simulink model "drone"  (Simulink 8.5)
settings: Solver=ode45  StartTime=0.0  StopTime=tsim  RelTol=1e-8  AbsTol=1e-12
undefined symbols (not defined in the file or in its folder): A, a_noise_seed, a_noise_var, a_scale, Cd, dx_init, enu2ecef, g, GPS_DT, GuideDt, h_noise_seed, h_noise_var, I, I_motor, IMU_DT, KaQ, KaR, KDhover, KIhover, Kir, KPhover, Kpr, Kpv, KQ, KR, KthQ, KthR, m, mag_bias, MAG_DT, mag_noise_seed, mag_noise_var, MaxPropRate, MaxPwmWidth, mean_a_bias, mean_w_bias, MinPwmWidth, mtow, P_init, Q, q0, qInit, R, r0, r1, r2, r3, r4, r_gps, RateToForce, Re, rho, Rmag, RunUpLimit, RunUpStartThrottle, tc, v0, v_noise_seed, v_noise_var, vc ... (+7)
libraries: simulink x13, SimLib x3
(part 1 of 2)
settings Model: Creator=Mike  LastModifiedBy=Walker  CovSFcnEnable=off
settings SolverCC: ZeroCrossControl=DisableAll
settings DebuggingCC: SolverPrmCheckMsg=warning  FcnCallInpInsideContextMsg=UseLocalSettings

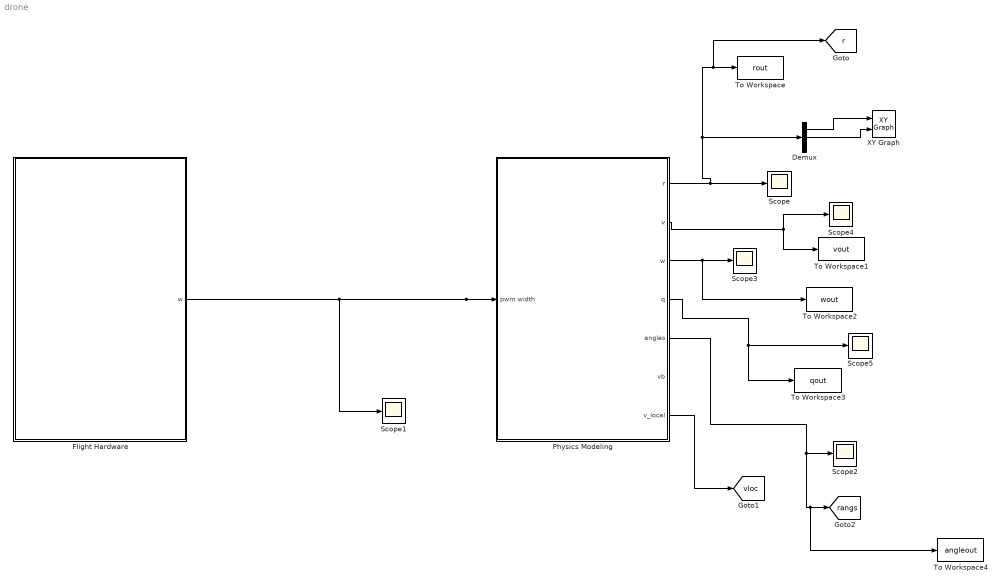
== system drone ==
  Demux : Demux  Outputs=3
  Flight Hardware : Subsystem
  Physics Modeling : Subsystem
  Scope{,1..5} (6 alike) : Scope
      Scope settings: TimeRange=50  YMin=-0.5  YMax=7
      Scope1 settings: TimeRange=30  YMin=1.5  YMax=1.975
      Scope2 settings: TimeRange=17  YMin=-200  YMax=200  SaveName=ScopeData5
      Scope3 settings: TimeRange=50  YMin=-1  YMax=1  SaveName=ScopeData13
      Scope4 settings: TimeRange=66.02  YMin=0  YMax=1.4  SaveName=ScopeData38
      Scope5 settings: TimeRange=100  YMin=0  YMax=1  SaveName=ScopeData96
  To Workspace : ToWorkspace  VariableName=rout  SampleTime=IMU_DT
  To Workspace1 : ToWorkspace  VariableName=vout  SampleTime=IMU_DT
  To Workspace2 : ToWorkspace  VariableName=wout  SampleTime=IMU_DT
  To Workspace3 : ToWorkspace  VariableName=qout  SampleTime=IMU_DT
  To Workspace4 : ToWorkspace  VariableName=angleout  SampleTime=IMU_DT
  XY Graph : simulink/Sinks/XY Graph  xmin=-20  xmax=20  ymin=-20  ymax=20  st=1
  tag scope: r=global, rangs=global, vloc=global
  wires:
  Flight Hardware/1(w) -> Scope1/1, Physics Modeling/1("pwm width ")
  Physics Modeling/1(r) -> Demux/1, To Workspace/1, [r], Scope/1
  Physics Modeling/5(angles) -> Scope2/1, To Workspace4/1, [rangs]
  Physics Modeling/3(w) -> Scope3/1, To Workspace2/1
  Physics Modeling/2(v) -> Scope4/1, To Workspace1/1
  Demux/1 -> XY Graph/1
  Demux/2 -> XY Graph/2
  Physics Modeling/4(q) -> To Workspace3/1, Scope5/1
  Physics Modeling/7(v_local) -> [vloc]

== system drone/Flight Hardware ==
  Scope2 : Scope
      settings: TimeRange=80  YMin=-1  YMax=6  SaveName=ScopeData80
  Sensor Model : Subsystem
  Unit Delay{,1,3..4} (4 alike) : UnitDelay  SampleTime=-1
  Unit Delay2 : UnitDelay  InitialCondition=[0 0 0 1]  SampleTime=-1
  Zero-Order Hold3 : ZeroOrderHold  SampleTime=IMU_DT
  control : Subsystem
  sample{1..6} (6 alike) : RateTransition  OutPortSampleTime=0.01
  state estimator1 : Subsystem
  w : Outport
  wires:
  Zero-Order Hold3/1 -> w/1
  control/1(rate blades) -> Zero-Order Hold3/1
  Sensor Model/2(w_b) -> sample6/1, state estimator1/2(w_b)
  [r] -> sample3/1
  [quat] -> sample4/1
  [V_uen] -> sample5/1
  Sensor Model/3(h) -> state estimator1/3(r1)
  [w_b] -> sample1/1
  Sensor Model/4(mag) -> state estimator1/4(mag)
  state estimator1/1(r) -> Unit Delay/1, Scope2/1
  Sensor Model/1(a_b) -> state estimator1/1(a_b), sample2/1
  state estimator1/2(qs) -> Unit Delay2/1
  state estimator1/3(v) -> Unit Delay1/1
  state estimator1/4(w) -> Unit Delay3/1
  state estimator1/5(a) -> Unit Delay4/1
  Unit Delay/1 -> control/1(r)
  Unit Delay2/1 -> control/2(q)
  Unit Delay1/1 -> control/3(VUEN)
  Unit Delay3/1 -> control/4(w)
  Unit Delay4/1 -> control/5(a_b)

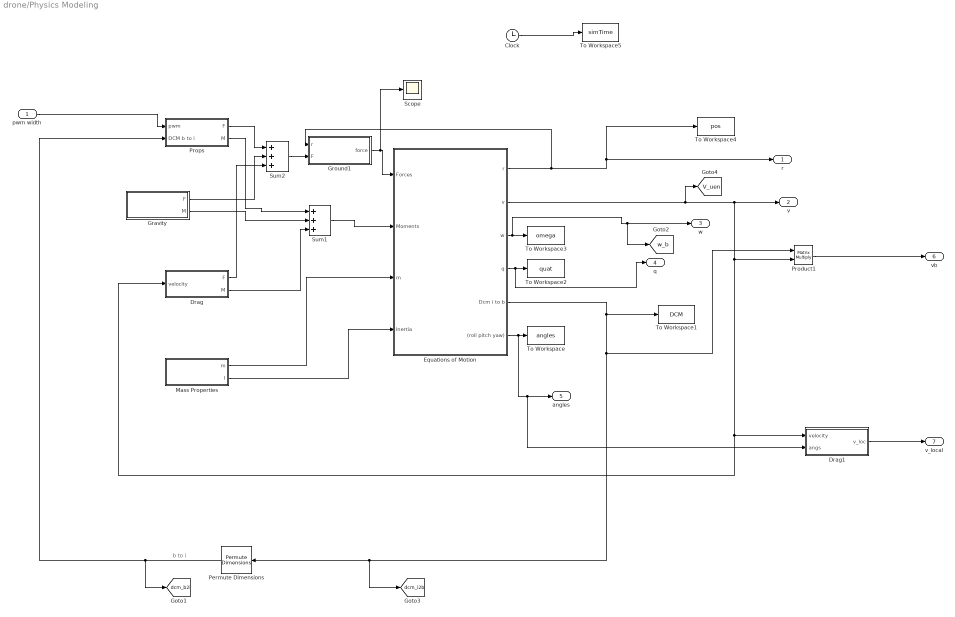
== system drone/Physics Modeling ==
  note: b to i
  "pwm width " : Inport
  Clock : Clock
  Drag : Subsystem
  Drag1 : Subsystem
  Equations of Motion : Subsystem
  Gravity : Subsystem
  Ground1 : Subsystem
  Mass Properties : Subsystem
  Permute Dimensions : PermuteDimensions
  Product1 : Product  Multiplication=Matrix(*)  RndMeth=Zero
  Props : Subsystem
  Scope : Scope
      settings: TimeRange=5.350553505535055  YMin=-4  SaveName=ScopeData58
  Sum1 : Sum  Inputs=+++
  Sum2 : Sum  Inputs=+++
  To Workspace : ToWorkspace  VariableName=angles  SampleTime=-1
  To Workspace1 : ToWorkspace  VariableName=DCM  SampleTime=-1
  To Workspace2 : ToWorkspace  VariableName=quat  SampleTime=-1
  To Workspace3 : ToWorkspace  VariableName=omega  SampleTime=-1
  To Workspace4 : ToWorkspace  VariableName=pos  SampleTime=-1
  To Workspace5 : ToWorkspace  VariableName=simTime  SampleTime=-1
  r : Outport
  v : Outport  Port=2
  w : Outport  Port=3
  q : Outport  Port=4
  angles : Outport  Port=5
  vb : Outport  Port=6
  v_local : Outport  Port=7
  tag scope: V_uen=global, dcm_b2i=global, dcm_i2b=global, w_b=global
  wires:
  Props/1(F) -> Sum2/1
  Gravity/1(F) -> Sum2/2
  Drag/1(F) -> Sum2/3
  Props/2(M) -> Sum1/1
  Gravity/2(M) -> Sum1/2
  Drag/2(M) -> Sum1/3
  Sum1/1 -> Equations of Motion/2(Moments)
  Mass Properties/1(m) -> Equations of Motion/3(m)
  Mass Properties/2(I) -> Equations of Motion/4(Inertia)
  "pwm width "/1 -> Props/1(pwm)
  Equations of Motion/2(v) -> Drag/1(velocity), Drag1/1(velocity), Product1/2, v/1, [V_uen]
  Equations of Motion/1(r) -> Ground1/1(r), To Workspace4/1, r/1
  Equations of Motion/6((roll pitch yaw)) -> To Workspace/1, angles/1, Drag1/2(angs)
  Equations of Motion/5(Dcm i to b) -> To Workspace1/1, Product1/1, Permute Dimensions/1, [dcm_i2b]
  Equations of Motion/4(q) -> To Workspace2/1, q/1
  Equations of Motion/3(w) -> To Workspace3/1, w/1, [w_b]
  Permute Dimensions/1 -> [dcm_b2i], Props/2("DCM b to i ")
  Product1/1 -> vb/1
  Drag1/1(v_loc) -> v_local/1
  Clock/1 -> To Workspace5/1
  Ground1/1(force) -> Scope/1, Equations of Motion/1(Forces)
  Sum2/1 -> Ground1/2(F)

== system drone/Flight Hardware/Sensor Model ==
  Acceleration model : Subsystem
  Angular Velocity Model : Subsystem
  Digital Clock2 : DigitalClock  SampleTime=IMU_DT
  GPS Model : Subsystem
  Mag Model1 : Subsystem
  To Workspace1 : ToWorkspace  VariableName=sensorMag  SampleTime=-1
  To Workspace3 : ToWorkspace  VariableName=sensorGyro  SampleTime=-1
  To Workspace4 : ToWorkspace  VariableName=imuTime  SampleTime=-1
  To Workspace5 : ToWorkspace  VariableName=MagTime  SampleTime=-1
  To Workspace6 : ToWorkspace  VariableName=GpsTime  SampleTime=-1
  To Workspace7 : ToWorkspace  VariableName=sensorAccel  SampleTime=-1
  sample1 : RateTransition  OutPortSampleTime=MAG_DT
  sample2 : RateTransition  OutPortSampleTime=GPS_DT
  a_b : Outport
  w_b : Outport  Port=2
  h : Outport  Port=3
  mag : Outport  Port=4
  wires:
  Acceleration model/1(Out1) -> a_b/1, To Workspace7/1
  Angular Velocity Model/1(Out1) -> To Workspace3/1, w_b/1
  GPS Model/1(h) -> h/1
  Mag Model1/1(mag field) -> To Workspace1/1, mag/1
  Digital Clock2/1 -> To Workspace4/1, sample1/1, sample2/1
  sample1/1 -> To Workspace5/1
  sample2/1 -> To Workspace6/1

== system drone/Flight Hardware/control ==
  note: x,y,z
  r : Inport
  q : Inport  Port=2
  VUEN : Inport  Port=3
  w : Inport  Port=4
  a_b : Inport  Port=5
  Autopilot : Subsystem
  Constant : Constant  Value=mtow  SampleTime=IMU_DT
  Fin MIx : Product  Multiplication=Matrix(*)  RndMeth=Zero  OutDataTypeStr=Inherit: Same as first input
  Guidance : Subsystem
  Mux : Mux  Inputs=2
  RateToPwm : Subsystem
  Scope : Scope
      settings: TimeRange=80  YMin=-400000  YMax=400000  SaveName=ScopeData33
  Scope1 : Scope
      settings: TimeRange=27.17391304347826  YMin=-0.08  YMax=0.09999999999999999  SaveName=ScopeData130
  Scope2 : Scope
      settings: TimeRange=27.17391304347826  YMin=-0.08  YMax=0.09999999999999999  SaveName=ScopeData28
  To Workspace1 : ToWorkspace  VariableName=mCmd  SampleTime=-1
  To Workspace2 : ToWorkspace  VariableName=ApFtot  SampleTime=IMU_DT
  To Workspace3 : ToWorkspace  VariableName=bladeCmdSim  SampleTime=-1
  rate blades : Outport
  wires:
  r/1 -> Guidance/1(r)
  Fin MIx/1 -> RateToPwm/1(In1), To Workspace3/1, Scope/1
  Constant/1 -> Fin MIx/1
  Autopilot/1(M) -> Mux/1, To Workspace1/1, Scope2/1
  Mux/1 -> Fin MIx/2
  w/1 -> Autopilot/4(w_m)
  q/1 -> Autopilot/1(q)
  a_b/1 -> Autopilot/3(a_m)
  Guidance/1(a cmd) -> Autopilot/2(a_cmd)
  Guidance/2(vcmd) -> Autopilot/5(Vcmd)
  VUEN/1 -> Guidance/2(v)
  RateToPwm/1(Out1) -> rate blades/1
  Guidance/3(" f tot") -> Autopilot/6(Ftot), To Workspace2/1
  Autopilot/2("Throttle Cmd ") -> Scope1/1, Mux/2

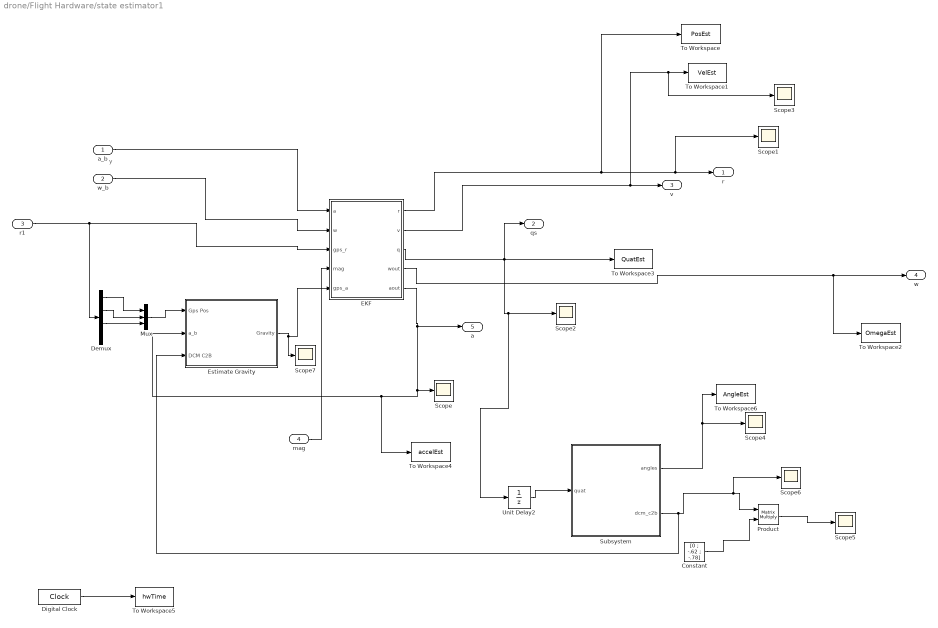
== system drone/Flight Hardware/state estimator1 ==
  note: y
  a_b : Inport
  w_b : Inport  Port=2
  r1 : Inport  Port=3
  mag : Inport  Port=4
  Constant : Constant  Value=[0 ; -.62 ; -.78]
  Demux : Demux
  Digital Clock : DigitalClock  SampleTime=IMU_DT
  EKF : Subsystem
  Estimate Gravity : Subsystem
  Mux : Mux  Inputs=3
  Product : Product  Multiplication=Matrix(*)
  Scope{,1..7} (8 alike) : Scope
      Scope settings: TimeRange=50  YMin=-1e+09  YMax=5e+09  SaveName=ScopeData29
      Scope1 settings: TimeRange=200  YMin=-1  YMax=8  SaveName=ScopeData90
      Scope2 settings: TimeRange=100  YMin=-1  YMax=0.2  SaveName=ScopeData89
      Scope3 settings: TimeRange=3.935786802879846  YMin=-0.3  YMax=0.3  SaveName=ScopeData92
      Scope4 settings: TimeRange=100  YMin=-20  YMax=120  SaveName=ScopeData110
      Scope5 settings: TimeRange=120  YMin=-1  YMax=1  SaveName=ScopeData111
      Scope6 settings: TimeRange=300  YMin=-0.8  YMax=0.8  SaveName=ScopeData112
      Scope7 settings: TimeRange=50  YMin=-5e+09  YMax=1e+09  SaveName=ScopeData9
  Subsystem : Subsystem
  To Workspace : ToWorkspace  VariableName=PosEst  SampleTime=-1
  To Workspace1 : ToWorkspace  VariableName=VelEst  SampleTime=-1
  To Workspace2 : ToWorkspace  VariableName=OmegaEst  SampleTime=-1
  To Workspace3 : ToWorkspace  VariableName=QuatEst  SampleTime=-1
  To Workspace4 : ToWorkspace  VariableName=accelEst  SampleTime=-1
  To Workspace5 : ToWorkspace  VariableName=hwTime  SampleTime=IMU_DT
  To Workspace6 : ToWorkspace  VariableName=AngleEst  SampleTime=-1
  Unit Delay2 : UnitDelay  InitialCondition=qInit  SampleTime=IMU_DT
  r : Outport
  qs : Outport  Port=2
  v : Outport  Port=3
  w : Outport  Port=4
  a : Outport  Port=5
  wires:
  EKF/3(q) -> qs/1, To Workspace3/1, Unit Delay2/1, Scope2/1
  EKF/1(r) -> To Workspace/1, r/1, Scope1/1
  EKF/2(v) -> v/1, Scope3/1, To Workspace1/1
  w_b/1 -> EKF/2(w)
  EKF/4(wout) -> To Workspace2/1, w/1
  r1/1 -> Demux/1, EKF/3(gps_r)
  mag/1 -> EKF/4(mag)
  Subsystem/1(angles) -> To Workspace6/1, Scope4/1
  Constant/1 -> Product/2
  Product/1 -> Scope5/1
  Mux/1 -> Estimate Gravity/1(Gps Pos)
  Demux/1 -> Mux/1
  Demux/2 -> Mux/2
  Demux/3 -> Mux/3
  Estimate Gravity/1(Gravity) -> Scope7/1, EKF/5(gps_a)
  Unit Delay2/1 -> Subsystem/1(quat)
  Subsystem/2(dcm_c2b) -> Estimate Gravity/3(DCM C2B), Scope6/1, Product/1
  a_b/1 -> EKF/1(a)
  EKF/5(aout) -> To Workspace4/1, Estimate Gravity/2(a_b), Scope/1, a/1
  Digital Clock/1 -> To Workspace5/1

== system drone/Physics Modeling/Drag ==
  velocity : Inport
  Abs : Abs
  Constant : Constant  Value=rho*Cd*A
  Gain : Gain  Gain=-0.5
  Product : Product  Inputs=***  RndMeth=Zero
  Scope : Scope
      settings: TimeRange=80  SaveName=ScopeData54
  assume cp = cm : Constant  Value=0
  F : Outport
  M : Outport  Port=2
  tag scope: faero_i=global
  wires:
  velocity/1 -> Abs/1, Gain/1
  Gain/1 -> Product/2
  Abs/1 -> Product/1
  Constant/1 -> Product/3
  assume cp = cm/1 -> M/1
  Product/1 -> F/1, [faero_i], Scope/1

== system drone/Physics Modeling/Drag1 ==
  velocity : Inport
  angs : Inport  Port=2
  Embedded MATLAB Function : MATLAB Function  TreatAsAtomicUnit=on
  Product : Product  Multiplication=Matrix(*)  RndMeth=Zero
  v_loc : Outport
  wires:
  velocity/1 -> Product/2
  Product/1 -> v_loc/1
  angs/1 -> Embedded MATLAB Function/1(u)
  Embedded MATLAB Function/1(y) -> Product/1

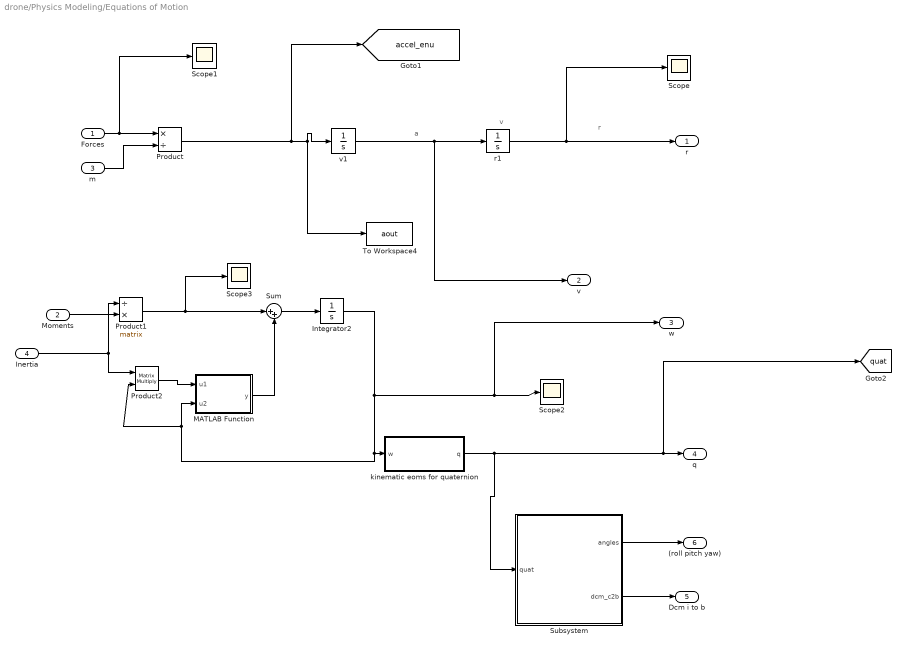
== system drone/Physics Modeling/Equations of Motion ==
  note: a
  note: v
  note: r
  Forces : Inport
  Moments : Inport  Port=2
  m : Inport  Port=3
  Inertia : Inport  Port=4
  Integrator2 : Integrator  InitialCondition=w0  AbsoluteTolerance=abstol
  MATLAB Function : MATLAB Function  TreatAsAtomicUnit=on
  Product : Product  Inputs=*/  RndMeth=Zero
  Product1 : Product  Inputs=/*  Multiplication=Matrix(*)  RndMeth=Zero
  Product2 : Product  Inputs=**  Multiplication=Matrix(*)  RndMeth=Zero
  Scope{,1..3} (4 alike) : Scope
      Scope settings: SaveName=ScopeData55
      Scope1 settings: TimeRange=100  SaveName=ScopeData56
      Scope2 settings: TimeRange=50  YMin=-2000  YMax=0  SaveName=ScopeData14
      Scope3 settings: TimeRange=50  YMin=-2000  YMax=0  SaveName=ScopeData37
  Subsystem : Subsystem
  Sum : Sum  Inputs=|++
  To Workspace4 : ToWorkspace  VariableName=aout  SampleTime=-1
  kinematic eoms for quaternion : Subsystem
  r1 : Integrator  InitialCondition=r0  AbsoluteTolerance=abstol
  v1 : Integrator  InitialCondition=v0  AbsoluteTolerance=abstol
  r : Outport
  v : Outport  Port=2
  w : Outport  Port=3
  q : Outport  Port=4
  Dcm i to b : Outport  Port=5
  (roll pitch yaw) : Outport  Port=6
  tag scope: accel_enu=global, quat=global
  wires:
  r1/1 -> Scope/1, r/1
  v1/1 -> r1/1, v/1
  Forces/1 -> Product/1, Scope1/1
  m/1 -> Product/2
  kinematic eoms for quaternion/1(q) -> Subsystem/1(quat), q/1, [quat]
  Subsystem/2(dcm_c2b) -> Dcm i to b/1
  Subsystem/1(angles) -> (roll pitch yaw)/1
  Inertia/1 -> Product1/1, Product2/1
  Moments/1 -> Product1/2
  Integrator2/1 -> Scope2/1, w/1, kinematic eoms for quaternion/1(w), MATLAB Function/2(u2), Product2/2
  Product2/1 -> MATLAB Function/1(u1)
  Sum/1 -> Integrator2/1
  Product1/1 -> Sum/1, Scope3/1
  MATLAB Function/1(y) -> Sum/2
  Product/1 -> [accel_enu], v1/1, To Workspace4/1

== system drone/Physics Modeling/Gravity ==
  Ground1 : Subsystem
  No horizontal : Gain  Gain=m
  Scope : Scope
      settings: SaveName=ScopeData57
  cg=cm in this problem : Constant  Value=0
  mg : Constant  Value=[0;0; -m*g ]
  F : Outport
  M : Outport  Port=2
  wires:
  cg=cm in this problem/1 -> M/1
  mg/1 -> F/1, Scope/1
  Ground1/1(accel) -> No horizontal/1

== system drone/Physics Modeling/Ground1 ==
  r : Inport
  F : Inport  Port=2
  Compare To Zero : simulink/Logic and Bit Operations/Compare To Zero  relop=<=  OutDataTypeStr=boolean  ZeroCross=off
  Constant : Constant  Value=0
  Constant1 : Constant  Value=0
  Demux : Demux  Outputs=3
  Saturation : Saturate  UpperLimit=inf  LowerLimit=0
  Scope{,1..3} (4 alike) : Scope
      Scope settings: YMin=-10  YMax=10  SaveName=ScopeData88
      Scope1 settings: TimeRange=20  YMin=0  YMax=3e-14  SaveName=ScopeData51
      Scope2 settings: YMin=-10  YMax=0  SaveName=ScopeData127
      Scope3 settings: YMin=9.5  YMax=20  SaveName=ScopeData128
  Sum : Sum  Inputs=|++
  Sum1 : Sum  Inputs=|+-
  Switch : Switch  Criteria=u2 > Threshold  Threshold=0.1
  Terminator : Terminator
  Terminator1 : Terminator
  force : Outport
  wires:
  r/1 -> Demux/1
  Demux/1 -> Terminator/1
  Demux/2 -> Terminator1/1
  Demux/3 -> Compare To Zero/1
  Compare To Zero/1 -> Switch/2
  Saturation/1 -> Switch/1, Scope3/1
  Switch/1 -> Sum/1
  Sum/1 -> Scope/1, force/1
  F/1 -> Scope2/1, Sum1/2, Sum/2
  Constant/1 -> Sum1/1
  Sum1/1 -> Saturation/1
  Constant1/1 -> Switch/3

== system drone/Physics Modeling/Mass Properties ==
  Constant : Constant  Value=m
  a : Constant  Value=I
  m : Outport
  I : Outport  Port=2
  tag scope: mass=global
  wires:
  a/1 -> I/1
  Constant/1 -> m/1, [mass]

== system drone/Physics Modeling/Props ==
  pwm : Inport
  "DCM b to i " : Inport  Port=2
  Gain : Gain
  Product : Product  Multiplication=Matrix(*)  OutDataTypeStr=Inherit: Inherit via back propagation  RndMeth=Nearest
  Rate to Force : Subsystem
  Rate to Force2 : Subsystem
  Scope{1..7} (7 alike) : Scope
      Scope1 settings: TimeRange=50  YMin=0  YMax=200  SaveName=ScopeData2
      Scope2 settings: YMin=-1  YMax=1  SaveName=ScopeData3
      Scope3 settings: TimeRange=50  YMin=-1.5  YMax=1.5  SaveName=ScopeData4
      Scope4 settings: TimeRange=6.110074626865668  YMin=-3.63961038961039e-009  YMax=-3.405844155844153e-009  SaveName=ScopeData11
      Scope5 settings: TimeRange=50  YMin=0  YMax=4e+14  SaveName=ScopeData9
      Scope6 settings: TimeRange=50  YMin=0  YMax=40  SaveName=ScopeData59
      Scope7 settings: TimeRange=0.2158273381295004  YMin=-1  YMax=1  SaveName=ScopeData62
  Sum : Sum
  Voltage to Rate : Subsystem
  F : Outport
  M : Outport  Port=2
  tag scope: fprop_i=global
  wires:
  pwm/1 -> Voltage to Rate/1(pwm width)
  Voltage to Rate/1(w) -> Rate to Force/1(w), Rate to Force2/1(w), Scope3/1
  Sum/1 -> Scope4/1, Gain/1
  Rate to Force/2(M) -> Sum/1, Scope2/1
  Rate to Force2/1(M) -> Sum/2, Scope1/1
  Product/1 -> [fprop_i], Scope6/1, F/1
  "DCM b to i "/1 -> Product/1, Scope7/1
  Rate to Force/1(Force) -> Product/2, Scope5/1
  Gain/1 -> M/1

== system drone/Flight Hardware/Sensor Model/Acceleration model ==
  Constant : Constant  Value=[0 0 g]
  Divide1 : Product  Inputs=**  Multiplication=Matrix(*)
  Quantizer : Quantizer  QuantizationInterval=AccelQuant
  Scope{1..3,5} (4 alike) : Scope
      Scope1 settings: TimeRange=30  YMin=0  YMax=40  SaveName=ScopeData46
      Scope2 settings: TimeRange=35  YMin=-2.5  YMax=40  SaveName=ScopeData47
      Scope3 settings: TimeRange=35  YMin=0  YMax=1  SaveName=ScopeData100
      Scope5 settings: TimeRange=49.99000000000001  YMin=9.763194444444443  YMax=9.821527777777776  SaveName=ScopeData101
  Sum : Sum  Inputs=+++
  To Workspace : ToWorkspace  VariableName=accel_measure  SampleTime=-1
  model measurment noise : Subsystem
  sample : RateTransition  X0=[0 0 g]  OutPortSampleTime=IMU_DT
  Out1 : Outport
  wires:
  Constant/1 -> Sum/2
  [accel_enu] -> Sum/1, Scope1/1
  sample/1 -> model measurment noise/1("true "), Scope2/1
  Divide1/1 -> sample/1
  Sum/1 -> Divide1/2, Scope5/1
  [dcm_i2b] -> Divide1/1, Scope3/1
  model measurment noise/1(noisy) -> Quantizer/1
  Quantizer/1 -> To Workspace/1, Out1/1

== system drone/Flight Hardware/Sensor Model/Angular Velocity Model ==
  Product : Product  Multiplication=Matrix(*)  RndMeth=Zero
  Quantizer : Quantizer  QuantizationInterval=GyroQuant
  Scope : Scope
      settings: TimeRange=30  YMin=-0.06  YMax=0.08  SaveName=ScopeData61
  Sum : Sum  Inputs=|++
  To Workspace1 : ToWorkspace  VariableName=omega_measure  SampleTime=-1
  earth rot rate (rads/sec)--assume at lat,log h (0,0,0) : Constant  Value=[0;0;0.00007272205]
  model measurment noise : Subsystem
  sample : RateTransition  OutPortSampleTime=IMU_DT
  Out1 : Outport
  wires:
  sample/1 -> model measurment noise/1("true ")
  earth rot rate (rads/sec)--assume at lat,log h (0,0,0)/1 -> Product/2
  [dcm_i2b] -> Product/1
  Product/1 -> ?
  [w_b] -> Sum/1
  Sum/1 -> sample/1
  model measurment noise/1(noisy) -> Quantizer/1
  Quantizer/1 -> To Workspace1/1, Scope/1, Out1/1

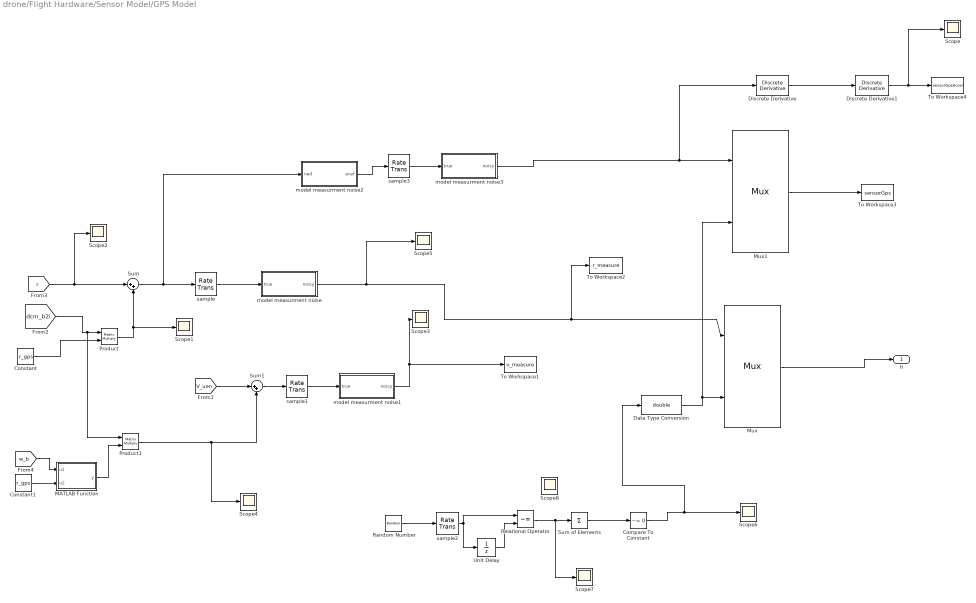
== system drone/Flight Hardware/Sensor Model/GPS Model ==
  Compare To Constant : simulink/Logic and Bit Operations/Compare To Constant  relop=~=  const=0  OutDataTypeStr=uint8  ZeroCross=off
  Constant : Constant  Value=r_gps
  Constant1 : Constant  Value=r_gps
  Data Type Conversion : DataTypeConversion  OutDataTypeStr=double
  Discrete Derivative : simulink/Discrete/Discrete Derivative  gainval=1  ICPrevScaledInput=0.0  InputProcessing=Inherited  OutMin=[]  OutMax=[]  OutDataType=fixdt(1, 16)  OutScaling=2^-10  DoSatur=off
  Discrete Derivative1 : simulink/Discrete/Discrete Derivative  gainval=1.0  ICPrevScaledInput=0  InputProcessing=Inherited  OutMin=[]  OutMax=[]  OutDataType=fixdt(1, 16)  OutScaling=2^-10  DoSatur=off
  MATLAB Function : MATLAB Function  TreatAsAtomicUnit=on
  Mux : Mux  Inputs=2
  Mux1 : Mux  Inputs=2
  Product : Product  Multiplication=Matrix(*)  RndMeth=Zero
  Product1 : Product  Multiplication=Matrix(*)  RndMeth=Zero
  Random Number : RandomNumber  Seed=1  SampleTime=GPS_DT
  Relational Operator : RelationalOperator  Operator=~=  OutDataTypeStr=boolean
  Scope{,1..8} (9 alike) : Scope
      Scope settings: SaveName=ScopeData49
      Scope1 settings: TimeRange=30  YMin=-1  YMax=1  SaveName=ScopeData98
      Scope2 settings: TimeRange=30  YMin=1  YMax=5.25  SaveName=ScopeData97
      Scope3 settings: TimeRange=30  YMin=-0.075  YMax=0.2  SaveName=ScopeData103
      Scope4 settings: TimeRange=30  YMin=-0.35  YMax=0.125  SaveName=ScopeData104
      Scope5 settings: TimeRange=30  YMin=3.5  YMax=11  SaveName=ScopeData94
      Scope6 settings: TimeRange=10  YMin=0.95  YMax=1.05  SaveName=ScopeData102
      Scope7 settings: TimeRange=0.4566066189408439  YMin=0  YMax=1  SaveName=ScopeData105
      Scope8 settings: TimeRange=10  YMin=-1  YMax=5.5  SaveName=ScopeData106
  Sum : Sum  Inputs=|++
  Sum of Elements : Sum  Inputs=+
  Sum1 : Sum  Inputs=|++
  To Workspace1 : ToWorkspace  VariableName=v_measure  SampleTime=GPS_DT
  To Workspace2 : ToWorkspace  VariableName=r_measure  SampleTime=IMU_DT
  To Workspace3 : ToWorkspace  VariableName=sensorGps  SampleTime=-1
  To Workspace4 : ToWorkspace  VariableName=sensorGpsAccel  SampleTime=IMU_DT
  Unit Delay : UnitDelay  InitialCondition=[0;0;0]  SampleTime=-1
  model measurment noise : Subsystem
  model measurment noise1 : Subsystem
  model measurment noise2 : Subsystem
  model measurment noise3 : Subsystem
  sample : RateTransition  OutPortSampleTime=GPS_DT
  sample1 : RateTransition  OutPortSampleTime=GPS_DT
  sample2 : RateTransition  OutPortSampleTime=IMU_DT
  sample3 : RateTransition  OutPortSampleTime=GPS_DT
  h : Outport  OutDataTypeStr=double
  wires:
  sample/1 -> model measurment noise/1("true ")
  sample1/1 -> model measurment noise1/1("true ")
  model measurment noise1/1(noisy) -> Scope3/1, To Workspace1/1
  Constant/1 -> Product/2
  [dcm_b2i] -> Product/1, Product1/1
  Sum/1 -> model measurment noise2/1("ned "), sample/1
  Product/1 -> Sum/2, Scope1/1
  [r] -> Sum/1, Scope2/1
  Sum1/1 -> sample1/1
  [V_uen] -> Sum1/1
  Constant1/1 -> MATLAB Function/2(u2)
  [w_b] -> MATLAB Function/1(u1)
  Product1/1 -> Sum1/2, Scope4/1
  model measurment noise/1(noisy) -> Scope5/1, Mux/1, To Workspace2/1
  Unit Delay/1 -> Relational Operator/2
  Relational Operator/1 -> Sum of Elements/1, Scope7/1
  Sum of Elements/1 -> Compare To Constant/1
  Compare To Constant/1 -> Scope6/1, Data Type Conversion/1
  sample2/1 -> Unit Delay/1, Relational Operator/1
  Mux/1 -> h/1
  MATLAB Function/1(y) -> Product1/2
  Data Type Conversion/1 -> Mux1/2, Mux/2
  Random Number/1 -> sample2/1
  model measurment noise2/1(ecef) -> sample3/1
  sample3/1 -> model measurment noise3/1("true ")
  model measurment noise3/1(noisy) -> Discrete Derivative/1, Mux1/1
  Mux1/1 -> To Workspace3/1
  Discrete Derivative/1 -> Discrete Derivative1/1
  Discrete Derivative1/1 -> Scope/1, To Workspace4/1

== system drone/Flight Hardware/Sensor Model/Mag Model1 ==
  Compare To Constant : simulink/Logic and Bit Operations/Compare To Constant  relop=~=  const=0  OutDataTypeStr=uint8  ZeroCross=off
  Data Type Conversion : DataTypeConversion  OutDataTypeStr=double
  Embedded MATLAB Function : MATLAB Function  TreatAsAtomicUnit=on
  Mux : Mux  Inputs=2
  Product : Product  Multiplication=Matrix(*)  RndMeth=Zero
  Relational Operator : RelationalOperator  Operator=~=  OutDataTypeStr=boolean
  Scope4 : Scope
      settings: TimeRange=300  YMin=-0.8  YMax=0.05  SaveName=ScopeData108
  Scope7 : Scope
      settings: TimeRange=0.4566066189408439  YMin=0  YMax=1  SaveName=ScopeData91
  Sum of Elements : Sum  Inputs=+
  To Workspace3 : ToWorkspace  VariableName=mag_measure  SampleTime=MAG_DT
  Unit Delay : UnitDelay  InitialCondition=[0;0;0]  SampleTime=-1
  model measurment noise1 : Subsystem
  sample1 : RateTransition  OutPortSampleTime=MAG_DT
  sample2 : RateTransition  OutPortSampleTime=IMU_DT
  mag field : Outport  OutDataTypeStr=double
  wires:
  sample1/1 -> model measurment noise1/1("true ")
  model measurment noise1/1(noisy) -> sample2/1, Scope4/1, Mux/1, To Workspace3/1
  Unit Delay/1 -> Relational Operator/2
  Relational Operator/1 -> Sum of Elements/1, Scope7/1
  Sum of Elements/1 -> Compare To Constant/1
  sample2/1 -> Unit Delay/1, Relational Operator/1
  Compare To Constant/1 -> Data Type Conversion/1
  Embedded MATLAB Function/1(Mhat) -> Product/2
  [dcm_i2b] -> Product/1
  Data Type Conversion/1 -> Mux/2
  Mux/1 -> mag field/1
  Product/1 -> sample1/1

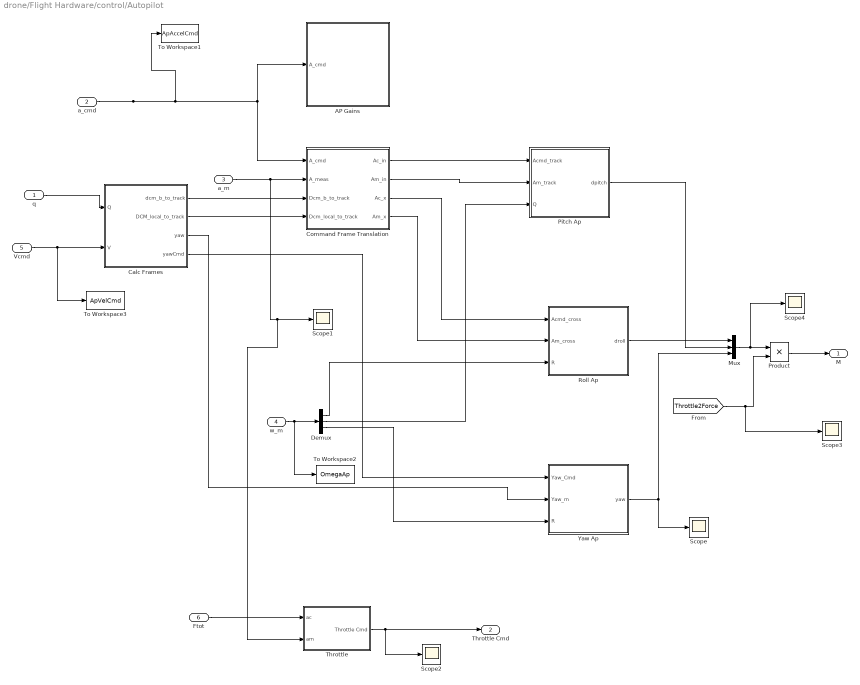
== system drone/Flight Hardware/control/Autopilot ==
  q : Inport
  a_cmd : Inport  Port=2
  a_m : Inport  Port=3
  w_m : Inport  Port=4
  Vcmd : Inport  Port=5
  Ftot : Inport  Port=6
  AP Gains : Subsystem
  Calc Frames : Subsystem
  Command Frame Translation : Subsystem
  Demux : Demux  Outputs=3
  Mux : Mux  Inputs=3
  Pitch Ap : Subsystem
  Product : Product
  Roll Ap : Subsystem
  Scope{,1..4} (5 alike) : Scope
      Scope settings: YMin=-0.00125  YMax=0.00075  SaveName=ScopeData6
      Scope1 settings: YMax=15  SaveName=ScopeData26
      Scope2 settings: TimeRange=100  YMin=0.95  YMax=1.05  SaveName=ScopeData36
      Scope3 settings: YMin=0.0238414  YMax=0.026351  SaveName=ScopeData125
      Scope4 settings: YMin=-6  YMax=7  SaveName=ScopeData126
  "Throttle " : Subsystem
  To Workspace1 : ToWorkspace  VariableName=ApAccelCmd  SampleTime=IMU_DT
  To Workspace2 : ToWorkspace  VariableName=OmegaAp  SampleTime=IMU_DT
  To Workspace3 : ToWorkspace  VariableName=ApVelCmd  SampleTime=IMU_DT
  Yaw Ap : Subsystem
  M : Outport
  "Throttle Cmd " : Outport  Port=2
  wires:
  w_m/1 -> To Workspace2/1, Demux/1
  a_m/1 -> "Throttle "/2(am), Scope1/1, Command Frame Translation/2(A_meas)
  Demux/2 -> Pitch Ap/3(Q)
  Command Frame Translation/2(Am_in) -> Pitch Ap/2(Am_track)
  Command Frame Translation/3(Ac_x) -> Roll Ap/1(Acmd_cross)
  Command Frame Translation/4(Am_x) -> Roll Ap/2(Am_cross)
  q/1 -> Calc Frames/1(Q)
  Calc Frames/1(dcm_b_to_track) -> Command Frame Translation/3(Dcm_b_to_track)
  Calc Frames/2(DCM_local_to_track) -> Command Frame Translation/4(Dcm_local_to_track)
  Calc Frames/3(yaw) -> Yaw Ap/2(Yaw_m)
  Yaw Ap/1(yaw) -> Mux/3, Scope/1
  Demux/1 -> Roll Ap/3(R)
  Demux/3 -> Yaw Ap/3(R)
  Vcmd/1 -> To Workspace3/1, Calc Frames/2(V)
  Roll Ap/1(droll) -> Mux/1
  Pitch Ap/1(dpitch) -> Mux/2
  Calc Frames/4(yawCmd) -> Yaw Ap/1(Yaw_Cmd)
  a_cmd/1 -> To Workspace1/1, AP Gains/1(A_cmd), Command Frame Translation/1(A_cmd)
  Ftot/1 -> "Throttle "/1(ac)
  Mux/1 -> Scope4/1, Product/1
  Product/1 -> M/1
  "Throttle "/1(Throttle Cmd) -> Scope2/1, "Throttle Cmd "/1
  Command Frame Translation/1(Ac_in) -> Pitch Ap/1(Acmd_track)
  [Throttle2Force] -> Scope3/1, Product/2

== system drone/Flight Hardware/control/Guidance ==
  r : Inport
  v : Inport  Port=2
  Digital Clock : DigitalClock  SampleTime=GuideDt
  Lookup Table : Lookup  InputValues=tc  Table=xc  LookUpMeth=Interpolation-Use End Values
  Lookup Table1 : Lookup  InputValues=tc  Table=yc  LookUpMeth=Interpolation-Use End Values
  Lookup Table2 : Lookup  InputValues=tc  Table=zc  LookUpMeth=Interpolation-Use End Values
  Lookup Table3 : Lookup  InputValues=tc  Table=vc(1,:)  LookUpMeth=Interpolation-Use End Values
  Lookup Table4 : Lookup  InputValues=tc  Table=vc(2,:)  LookUpMeth=Interpolation-Use End Values
  Mux1 : Mux  Inputs=2
  Mux2 : Mux  Inputs=3
  Rate Transition : RateTransition  OutPortSampleTime=GuideDt
  Rate Transition1 : RateTransition  OutPortSampleTime=GuideDt
  Scope2 : Scope
      settings: TimeRange=300  YMin=0  YMax=0.12  SaveName=ScopeData27
  Scope3 : Scope
      settings: TimeRange=100  YMin=-1  YMax=1  SaveName=ScopeData7
  To Workspace1 : ToWorkspace  VariableName=vCmd  SampleTime=-1
  To Workspace2 : ToWorkspace  VariableName=aCmd  SampleTime=-1
  To Workspace3 : ToWorkspace  VariableName=fTot  SampleTime=-1
  To Workspace4 : ToWorkspace  VariableName=guideTime  SampleTime=-1
  To Workspace5 : ToWorkspace  VariableName=guidePos  SampleTime=-1
  To Workspace6 : ToWorkspace  VariableName=guideVel  SampleTime=-1
  v1 cmd : Subsystem
  a cmd : Outport
  vcmd : Outport  Port=2
  " f tot" : Outport  Port=3
  tag scope: acmd_true=global
  wires:
  Digital Clock/1 -> To Workspace4/1, Lookup Table1/1, Lookup Table/1, Lookup Table2/1, Lookup Table3/1, Lookup Table4/1
  Lookup Table2/1 -> Scope3/1, Mux2/3
  Lookup Table3/1 -> Mux1/1
  Lookup Table4/1 -> Mux1/2
  Mux1/1 -> vcmd/1, To Workspace1/1, Scope2/1, v1 cmd/4(vc)
  Lookup Table1/1 -> Mux2/2
  Lookup Table/1 -> Mux2/1
  Mux2/1 -> v1 cmd/3(rc)
  v1 cmd/1(acmd) -> [acmd_true], To Workspace2/1, a cmd/1
  v1 cmd/2(f tot) -> To Workspace3/1, " f tot"/1
  r/1 -> Rate Transition/1
  Rate Transition/1 -> To Workspace5/1, v1 cmd/1(r)
  v/1 -> Rate Transition1/1
  Rate Transition1/1 -> To Workspace6/1, v1 cmd/2(v)

== system drone/Flight Hardware/control/RateToPwm ==
  In1 : Inport
  Abs : Abs
  Constant : Constant  Value=MinPwmWidth
  Gain : Gain  Gain=(MaxPwmWidth - MinPwmWidth)
  Saturation : Saturate  UpperLimit=MaxPwmWidth  LowerLimit=MinPwmWidth
  Sum : Sum  Inputs=|++
  Out1 : Outport
  wires:
  In1/1 -> Abs/1
  Abs/1 -> Gain/1
  Gain/1 -> Sum/1
  Constant/1 -> Sum/2
  Saturation/1 -> Out1/1
  Sum/1 -> Saturation/1

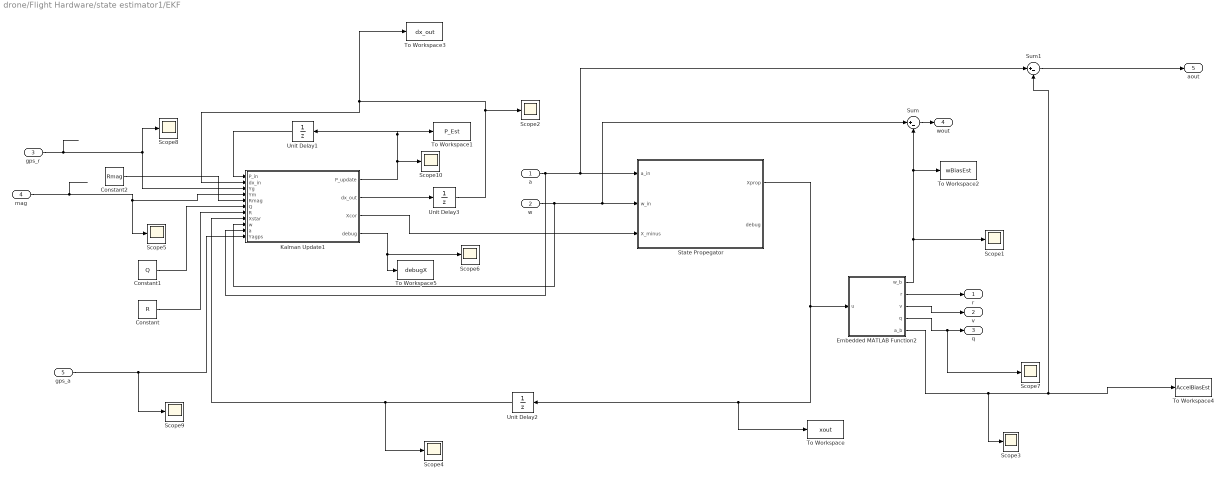
== system drone/Flight Hardware/state estimator1/EKF ==
  a : Inport
  w : Inport  Port=2
  gps_r : Inport  Port=3
  mag : Inport  Port=4
  gps_a : Inport  Port=5
  Constant : Constant  Value=R  SampleTime=IMU_DT
  Constant1 : Constant  Value=Q  SampleTime=IMU_DT
  Constant2 : Constant  Value=Rmag  SampleTime=IMU_DT
  Embedded MATLAB Function2 : MATLAB Function  TreatAsAtomicUnit=on
  Kalman Update1 : MATLAB Function  TreatAsAtomicUnit=on
  Scope{1..10} (10 alike) : Scope
      Scope1 settings: TimeRange=100  YMin=-0.03  YMax=0.04  SaveName=ScopeData93
      Scope10 settings: TimeRange=300  YMin=-0.0007  YMax=0.0006  SaveName=ScopeData116
      Scope2 settings: TimeRange=10  YMin=-900000  YMax=100000  SaveName=ScopeData107
      Scope3 settings: TimeRange=100  YMin=-0.3  YMax=0.5  SaveName=ScopeData63
      Scope4 settings: TimeRange=100  YMin=-0.5  YMax=6.5  SaveName=ScopeData95
      Scope5 settings: TimeRange=100  YMin=-45  YMax=25  SaveName=ScopeData99
      Scope6 settings: TimeRange=40  YMin=-0.8  YMax=0.05  SaveName=ScopeData109
      Scope7 settings: TimeRange=100  YMin=-0.05  YMax=1  SaveName=ScopeData113
      Scope8 settings: TimeRange=0.3874475772223365  YMin=0  YMax=1  SaveName=ScopeData32
      Scope9 settings: TimeRange=9.365558912386732  YMin=-100  YMax=80  SaveName=ScopeData10
  State Propegator : MATLAB Function  TreatAsAtomicUnit=on
  Sum : Sum  Inputs=|+-
  Sum1 : Sum  Inputs=|+-
  To Workspace : ToWorkspace  VariableName=xout  SampleTime=-1
  To Workspace1 : ToWorkspace  VariableName=P_Est  SampleTime=-1
  To Workspace2 : ToWorkspace  VariableName=wBiasEst  SampleTime=-1
  To Workspace3 : ToWorkspace  VariableName=dx_out  SampleTime=-1
  To Workspace4 : ToWorkspace  VariableName=AccelBiasEst  SampleTime=-1
  To Workspace5 : ToWorkspace  VariableName=debugX  SampleTime=-1
  Unit Delay1 : UnitDelay  InitialCondition=P_init  SampleTime=IMU_DT
  Unit Delay2 : UnitDelay  InitialCondition=x_init  SampleTime=IMU_DT
  Unit Delay3 : UnitDelay  InitialCondition=dx_init  SampleTime=IMU_DT
  r : Outport  SampleTime=IMU_DT
  v : Outport  Port=2  SampleTime=IMU_DT
  q : Outport  Port=3  SampleTime=IMU_DT
  wout : Outport  Port=4  SampleTime=IMU_DT
  aout : Outport  Port=5  SampleTime=IMU_DT
  wires:
  Unit Delay1/1 -> Kalman Update1/1(P_in)
  Kalman Update1/1(P_update) -> Scope10/1, Unit Delay1/1, To Workspace1/1
  a/1 -> Kalman Update1/10(a), Sum1/1, State Propegator/1(a_in)
  w/1 -> Kalman Update1/9(w), State Propegator/2(w_in), Sum/1
  gps_r/1 -> Kalman Update1/3(Yg), Scope8/1
  Constant/1 -> Kalman Update1/7(R)
  Constant1/1 -> Kalman Update1/6(Q)
  Embedded MATLAB Function2/1(w_b) -> To Workspace2/1, Sum/2, Scope1/1
  Sum/1 -> wout/1
  Embedded MATLAB Function2/2(r) -> r/1
  Embedded MATLAB Function2/3(v) -> v/1
  Embedded MATLAB Function2/4(q) -> Scope7/1, q/1
  Embedded MATLAB Function2/5(a_b) -> Sum1/2, To Workspace4/1, Scope3/1
  Kalman Update1/2(dx_out) -> Unit Delay3/1
  Unit Delay3/1 -> Kalman Update1/2(dx_in), To Workspace3/1, Scope2/1
  State Propegator/1(Xprop) -> Embedded MATLAB Function2/1(u), Unit Delay2/1, To Workspace/1
  Kalman Update1/3(Xcor) -> State Propegator/3(X_minus)
  Unit Delay2/1 -> Kalman Update1/8(Xstar), Scope4/1
  mag/1 -> Kalman Update1/4(Ym), Scope5/1
  Constant2/1 -> Kalman Update1/5(Rmag)
  Kalman Update1/4(debug) -> To Workspace5/1, Scope6/1
  Sum1/1 -> aout/1
  gps_a/1 -> Scope9/1, Kalman Update1/11(Yagps)

== system drone/Flight Hardware/state estimator1/Estimate Gravity ==
  Gps Pos : Inport
  a_b : Inport  Port=2
  DCM C2B : Inport  Port=3
  Discrete Derivative : simulink/Discrete/Discrete Derivative  gainval=1  ICPrevScaledInput=0.0  InputProcessing=Inherited  OutMin=[]  OutMax=[]  OutDataType=fixdt(1, 16)  OutScaling=2^-10  DoSatur=off
  Discrete Derivative1 : simulink/Discrete/Discrete Derivative  gainval=1.0  ICPrevScaledInput=0  InputProcessing=Inherited  OutMin=[]  OutMax=[]  OutDataType=fixdt(1, 16)  OutScaling=2^-10  DoSatur=off
  Product : Product  Multiplication=Matrix(*)
  Scope{1..7} (7 alike) : Scope
      Scope1 settings: TimeRange=50  YMin=-10  YMax=2  SaveName=ScopeData12
      Scope2 settings: TimeRange=50  YMin=-12.5  YMax=12.5  SaveName=ScopeData13
      Scope3 settings: TimeRange=50  YMin=-12.5  YMax=12.5  SaveName=ScopeData14
      Scope4 settings: TimeRange=50  YMin=-1.5  YMax=0.5  SaveName=ScopeData15
      Scope5 settings: TimeRange=50  YMin=-12.5  YMax=12.5  SaveName=ScopeData16
      Scope6 settings: TimeRange=10  YMin=-12.5  YMax=12.5  SaveName=ScopeData87
      Scope7 settings: TimeRange=10  YMin=-300  YMax=200  SaveName=ScopeData11
  Sum : Sum  Inputs=|-+
  Gravity : Outport
  wires:
  Product/1 -> Sum/2, Scope7/1
  Gps Pos/1 -> Discrete Derivative/1, Scope3/1
  Discrete Derivative/1 -> Scope6/1, Discrete Derivative1/1
  Discrete Derivative1/1 -> Product/2, Scope4/1
  a_b/1 -> Sum/1, Scope5/1
  DCM C2B/1 -> Product/1
  Sum/1 -> Gravity/1, Scope1/1

== system drone/Flight Hardware/state estimator1/Subsystem ==
  note: Based on Prof Howell AAE 440 Notes
  note: C is row notation so transpose it!
  quat : Inport
  Permute Dimensions : PermuteDimensions
  solve direction cosine matrix : Subsystem
  angles : Outport
  dcm_c2b : Outport  Port=2
  wires:
  quat/1 -> solve direction cosine matrix/1(quat)
  solve direction cosine matrix/2(roll pitch yaw) -> angles/1
  solve direction cosine matrix/1(C) -> Permute Dimensions/1
  Permute Dimensions/1 -> dcm_c2b/1

== system drone/Physics Modeling/Equations of Motion/Subsystem ==
  note: Based on Prof Howell AAE 440 Notes
  note: C is row notation so transpose it!
  quat : Inport
  Permute Dimensions : PermuteDimensions
  solve direction cosine matrix : Subsystem
  angles : Outport
  dcm_c2b : Outport  Port=2
  wires:
  quat/1 -> solve direction cosine matrix/1(quat)
  solve direction cosine matrix/2(roll pitch yaw) -> angles/1
  solve direction cosine matrix/1(C) -> Permute Dimensions/1
  Permute Dimensions/1 -> dcm_c2b/1

== system drone/Physics Modeling/Equations of Motion/kinematic eoms for quaternion ==
  note: get these from notes
  note: w c2b
  w : Inport
  Demux : Demux  Outputs=3
  Demux1 : Demux
  Integrator : Integrator  InitialCondition=q0  AbsoluteTolerance=abstol  IgnoreLimit=on
  Mux : Mux  Inputs=7
  Mux1 : Mux
  Scope : Scope
      settings: SaveName=ScopeData60
  To Workspace2 : ToWorkspace  VariableName=qdots  SampleTime=-1
  q1dot : Fcn  Expr=.5*( u[5]*(u[3]) - u[6]*u[2] +u[7]*u[1])
  q2dot : Fcn  Expr=.5*(u[6]*u[1] + u[7]*u[2] -u[4]*(u[3]))
  q3dot : Fcn  Expr=.5*(u[7]*(u[3])+u[4]*u[2] - u[5]*u[1])
  q4dot : Fcn  Expr=.5*(-u[4]*u[1] - u[5]*u[2] - u[6]*(u[3]))
  q : Outport
  wires:
  Mux1/1 -> Integrator/1, To Workspace2/1
  Integrator/1 -> Demux1/1, q/1, Scope/1
  q4dot/1 -> Mux1/4
  q3dot/1 -> Mux1/3
  q2dot/1 -> Mux1/2
  q1dot/1 -> Mux1/1
  Mux/1 -> q1dot/1, q2dot/1, q3dot/1, q4dot/1
  w/1 -> Demux/1
  Demux/1 -> Mux/1
  Demux/2 -> Mux/2
  Demux/3 -> Mux/3
  Demux1/1 -> Mux/4
  Demux1/2 -> Mux/5
  Demux1/3 -> Mux/6
  Demux1/4 -> Mux/7

== system drone/Physics Modeling/Gravity/Ground1 ==
  r : Inport
  G : Inport  Port=2
  Compare To Zero : simulink/Logic and Bit Operations/Compare To Zero  relop=<=  OutDataTypeStr=boolean  ZeroCross=off
  Demux : Demux  Outputs=3
  No horizontal : Gain  Gain=[0 0 1]
  Saturation : Saturate  UpperLimit=[0 0 inf]  LowerLimit=[0 0 0]
  Scope : Scope
      settings: YMin=-0.0014  YMax=0  SaveName=ScopeData88
  Scope1 : Scope
      settings: TimeRange=20  YMin=0  YMax=3e-14  SaveName=ScopeData51
  Switch : Switch  Criteria=u2 > Threshold  Threshold=0.1
  Terminator : Terminator
  Terminator1 : Terminator
  accel : Outport
  wires:
  r/1 -> Demux/1
  Demux/1 -> Terminator/1
  Demux/2 -> Terminator1/1
  Demux/3 -> Compare To Zero/1
  G/1 -> No horizontal/1, Scope1/1, Switch/3
  Compare To Zero/1 -> Switch/2
  Switch/1 -> Scope/1, accel/1
  No horizontal/1 -> Saturation/1
  Saturation/1 -> Switch/1

== system drone/Physics Modeling/Props/Rate to Force ==
  note: F
  w : Inport
  Abs : Abs
  Demux : Demux
  Gain1 : Gain  Gain=RateToForce
  Scope3 : Scope
      settings: TimeRange=50  YMin=2.32987  YMax=2.57513  SaveName=ScopeData8
  Sum : Sum  Inputs=++++
  location moment : Subsystem
  location moment1 : Subsystem
  location moment2 : Subsystem
  location moment3 : Subsystem
  location moment4 : Subsystem
  Force : Outport
  M : Outport  Port=2
  wires:
  location moment/1(M) -> M/1
  Sum/1 -> Force/1
  location moment1/1(F1) -> Sum/1, location moment/1(F1)
  location moment2/1(F1) -> Sum/2, location moment/2(F2)
  location moment3/1(F1) -> Sum/3, location moment/3(F3)
  location moment4/1(F1) -> Sum/4, location moment/4(F4)
  Demux/1 -> location moment1/1(F)
  Demux/2 -> location moment2/1(F)
  Demux/3 -> location moment3/1(F)
  Demux/4 -> location moment4/1(F)
  Abs/1 -> Demux/1, Scope3/1
  w/1 -> Gain1/1
  Gain1/1 -> Abs/1

== system drone/Physics Modeling/Props/Rate to Force2 ==
  w : Inport
  Demux : Demux
  Gain : Gain  Gain=I_motor
  Motor 1 : Subsystem
  Motor 2 : Subsystem
  Motor 3 : Subsystem
  Motor 4 : Subsystem
  Sum : Sum  Inputs=++++
  M : Outport
  wires:
  w/1 -> Gain/1
  Gain/1 -> Demux/1
  Demux/1 -> Motor 1/1(w1)
  Demux/2 -> Motor 2/1(w2)
  Demux/4 -> Motor 4/1(w4)
  Motor 3/1(M) -> Sum/3
  Motor 4/1(M) -> Sum/4
  Motor 2/1(M) -> Sum/2
  Motor 1/1(M) -> Sum/1
  Sum/1 -> M/1
  Demux/3 -> Motor 3/1(w3)

== system drone/Physics Modeling/Props/Voltage to Rate ==
  pwm width : Inport
  Constant : Constant  Value=MinPwmWidth
  Gain : Gain  Gain=1/(MaxPwmWidth - MinPwmWidth)
  Gain1 : Gain  Gain=MaxPropRate
  Rotation Direction : Gain  Gain=[1 -1 1 -1]
  Sum : Sum  Inputs=|+-
  w : Outport
  wires:
  Constant/1 -> Sum/2
  Sum/1 -> Gain/1
  Rotation Direction/1 -> w/1
  pwm width/1 -> Sum/1
  Gain1/1 -> Rotation Direction/1
  Gain/1 -> Gain1/1

== system drone/Flight Hardware/Sensor Model/Acceleration model/model measurment noise ==
  "true " : Inport
  Random Number : RandomNumber  Mean=mean_a_bias  Variance=a_noise_var  Seed=a_noise_seed  SampleTime=IMU_DT
  Scope : Scope
      settings: TimeRange=30  YMin=-0.3  YMax=0.4  SaveName=ScopeData44
  Sum : Sum  Inputs=|++
  noisy : Outport
  wires:
  Random Number/1 -> Scope/1, Sum/2
  "true "/1 -> Sum/1
  Sum/1 -> noisy/1

== system drone/Flight Hardware/Sensor Model/Angular Velocity Model/model measurment noise ==
  "true " : Inport
  Random Number : RandomNumber  Mean=mean_w_bias  Variance=w_noise_var  Seed=w_noise_seed  SampleTime=IMU_DT
  Scope : Scope
      settings: TimeRange=60  YMin=-0.4  YMax=0.45  SaveName=ScopeData43
  Sum : Sum  Inputs=|++
  noisy : Outport
  wires:
  Random Number/1 -> Scope/1, Sum/2
  "true "/1 -> Sum/1
  Sum/1 -> noisy/1

== system drone/Flight Hardware/Sensor Model/GPS Model/model measurment noise ==
  "true " : Inport
  Discrete Derivative : simulink/Discrete/Discrete Derivative  gainval=1  ICPrevScaledInput=0.0  InputProcessing=Inherited  OutMin=[]  OutMax=[]  OutDataType=fixdt(1, 16)  OutScaling=2^-10  DoSatur=off
  Discrete Derivative1 : simulink/Discrete/Discrete Derivative  gainval=1.0  ICPrevScaledInput=0  InputProcessing=Inherited  OutMin=[]  OutMax=[]  OutDataType=fixdt(1, 16)  OutScaling=2^-10  DoSatur=off
  Random Number : RandomNumber  Variance=h_noise_var  Seed=h_noise_seed  SampleTime=GPS_DT
  Scope{,3..4,6} (4 alike) : Scope
      Scope settings: YMin=-0.15  YMax=0.15  SaveName=ScopeData43
      Scope3 settings: TimeRange=50  YMin=-12.5  YMax=12.5  SaveName=ScopeData73
      Scope4 settings: TimeRange=50  SaveName=ScopeData123
      Scope6 settings: TimeRange=10  YMin=-12.5  YMax=12.5  SaveName=ScopeData124
  Sum : Sum  Inputs=|++  AccumDataTypeStr=double
  noisy : Outport
  wires:
  "true "/1 -> Sum/1
  Sum/1 -> noisy/1
  Random Number/1 -> Discrete Derivative/1, Scope3/1, Scope/1, Sum/2
  Discrete Derivative/1 -> Scope6/1, Discrete Derivative1/1
  Discrete Derivative1/1 -> Scope4/1

== system drone/Flight Hardware/Sensor Model/GPS Model/model measurment noise1 ==
  "true " : Inport
  Random Number : RandomNumber  Variance=v_noise_var  Seed=v_noise_seed  SampleTime=GPS_DT
  Scope : Scope
      settings: SaveName=ScopeData43
  Sum : Sum  Inputs=|++  AccumDataTypeStr=double  OutDataTypeStr=Inherit: Same as first input
  noisy : Outport
  wires:
  Random Number/1 -> Scope/1, Sum/2
  "true "/1 -> Sum/1
  Sum/1 -> noisy/1

== system drone/Flight Hardware/Sensor Model/GPS Model/model measurment noise2 ==
  "ned " : Inport
  Constant : Constant  Value=enu2ecef
  Constant1 : Constant  Value=[0;0;Re]
  Divide : Product  Inputs=**  Multiplication=Matrix(*)
  Sum : Sum  Inputs=|++
  ecef : Outport
  wires:
  Constant/1 -> Divide/1
  Constant1/1 -> Sum/2
  "ned "/1 -> Sum/1
  Sum/1 -> Divide/2
  Divide/1 -> ecef/1

== system drone/Flight Hardware/Sensor Model/GPS Model/model measurment noise3 ==
  "true " : Inport
  Random Number : RandomNumber  Variance=h_noise_var  Seed=h_noise_seed  SampleTime=GPS_DT
  Scope : Scope
      settings: SaveName=ScopeData43
  Sum : Sum  Inputs=|++  AccumDataTypeStr=double
  noisy : Outport
  wires:
  Random Number/1 -> Scope/1, Sum/2
  "true "/1 -> Sum/1
  Sum/1 -> noisy/1

== system drone/Flight Hardware/Sensor Model/Mag Model1/model measurment noise1 ==
  "true " : Inport
  Random Number : RandomNumber  Mean=mag_bias  Variance=mag_noise_var  Seed=mag_noise_seed  SampleTime=MAG_DT
  Scope : Scope
      settings: TimeRange=300  SaveName=ScopeData43
  Sum : Sum  Inputs=|++
  noisy : Outport
  wires:
  Random Number/1 -> Scope/1, Sum/2
  "true "/1 -> Sum/1
  Sum/1 -> noisy/1

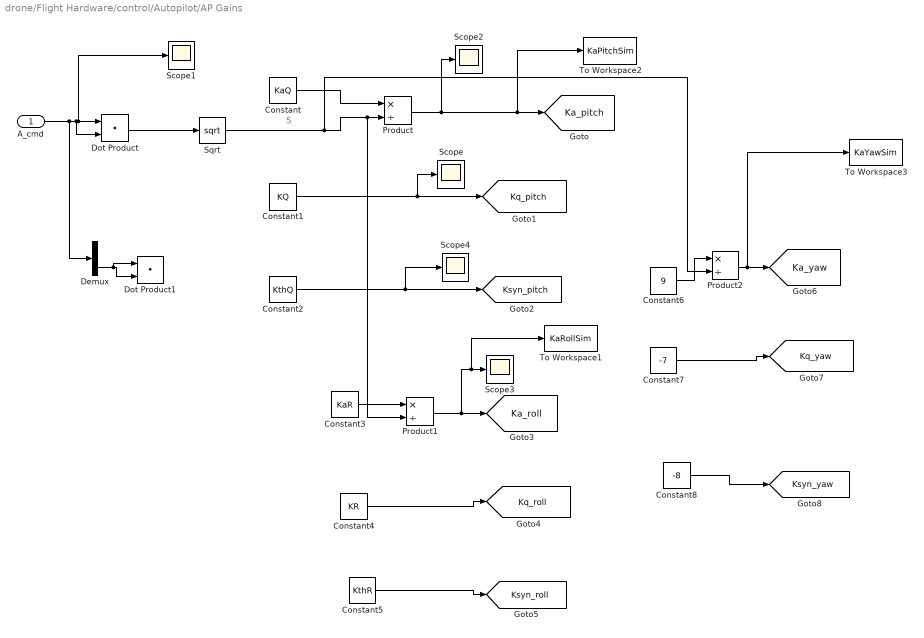
== system drone/Flight Hardware/control/Autopilot/AP Gains ==
  note: 5
  A_cmd : Inport
  Constant : Constant  Value=KaQ
  Constant1 : Constant  Value=KQ
  Constant2 : Constant  Value=KthQ
  Constant3 : Constant  Value=KaR
  Constant4 : Constant  Value=KR
  Constant5 : Constant  Value=KthR
  Constant6 : Constant  Value=9
  Constant7 : Constant  Value=-7
  Constant8 : Constant  Value=-8
  Demux : Demux  Outputs=3
  Dot Product : DotProduct  InputSameDT=on  OutDataTypeStr=Inherit: Inherit via internal rule
  Dot Product1 : DotProduct  InputSameDT=on  OutDataTypeStr=Inherit: Inherit via internal rule
  Product : Product  Inputs=*/
  Product1 : Product  Inputs=*/
  Product2 : Product  Inputs=*/
  Scope{,1..4} (5 alike) : Scope
      Scope settings: SaveName=ScopeData21
      Scope1 settings: YMin=0  YMax=15  SaveName=ScopeData35
      Scope2 settings: TimeRange=25  YMin=101.55  YMax=101.8  SaveName=ScopeData71
      Scope3 settings: TimeRange=25  YMin=0  YMax=23187.5  SaveName=ScopeData76
      Scope4 settings: SaveName=ScopeData118
  Sqrt : Sqrt  SaturateOnIntegerOverflow=on
  To Workspace1 : ToWorkspace  VariableName=KaRollSim  SampleTime=-1
  To Workspace2 : ToWorkspace  VariableName=KaPitchSim  SampleTime=-1
  To Workspace3 : ToWorkspace  VariableName=KaYawSim  SampleTime=-1
  tag scope: Ka_pitch=global, Ka_roll=global, Ka_yaw=global, Kq_pitch=global, Kq_roll=global, Kq_yaw=global, Ksyn_pitch=global, Ksyn_roll=global, Ksyn_yaw=global
  wires:
  A_cmd/1 -> Demux/1, Dot Product/1, Scope1/1, Dot Product/2
  Constant1/1 -> Scope/1, [Kq_pitch]
  Sqrt/1 -> Product2/2, Product1/2, Product/2
  Constant/1 -> Product/1
  Constant3/1 -> Product1/1
  Constant4/1 -> [Kq_roll]
  Constant5/1 -> [Ksyn_roll]
  Constant8/1 -> [Ksyn_yaw]
  Constant7/1 -> [Kq_yaw]
  Product2/1 -> To Workspace3/1, [Ka_yaw]
  Constant6/1 -> Product2/1
  Demux/3 -> Dot Product1/1, Dot Product1/2
  Dot Product/1 -> Sqrt/1
  Product/1 -> To Workspace2/1, [Ka_pitch], Scope2/1
  Product1/1 -> To Workspace1/1, Scope3/1, [Ka_roll]
  Constant2/1 -> Scope4/1, [Ksyn_pitch]

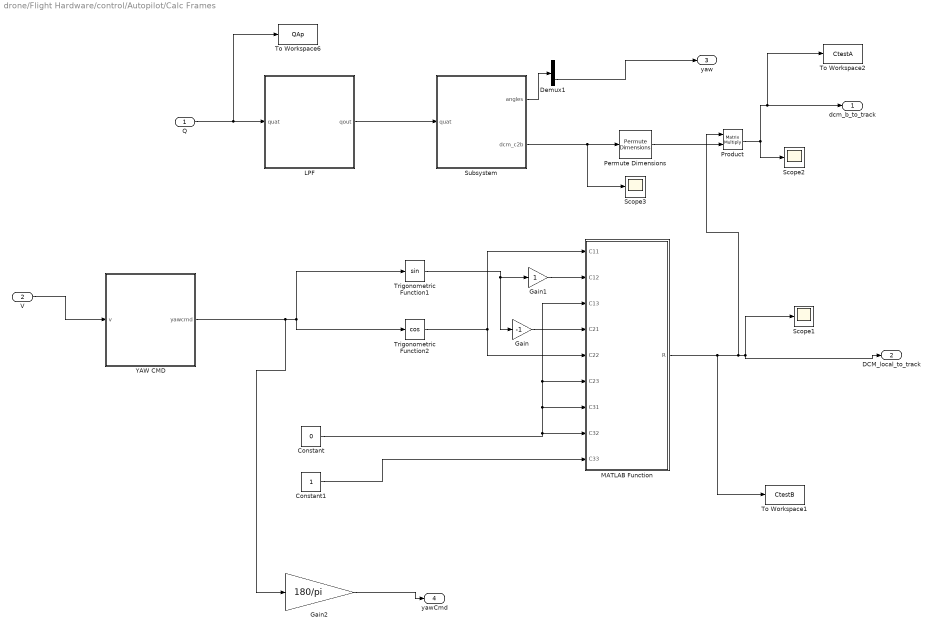
== system drone/Flight Hardware/control/Autopilot/Calc Frames ==
  Q : Inport
  V : Inport  Port=2
  Constant : Constant  Value=0  SampleTime=IMU_DT
  Constant1 : Constant  SampleTime=IMU_DT
  Demux1 : Demux  Outputs=3
  Gain : Gain  Gain=-1
  Gain1 : Gain
  Gain2 : Gain  Gain=180/pi  OutDataTypeStr=Inherit: Inherit via back propagation
  LPF : Subsystem
  MATLAB Function : MATLAB Function  TreatAsAtomicUnit=on  SystemSampleTime=IMU_DT
  Permute Dimensions : PermuteDimensions
  Product : Product  Multiplication=Matrix(*)
  Scope1 : Scope
      settings: YMin=-1  YMax=1  SaveName=ScopeData41
  Scope2 : Scope
      settings: SaveName=ScopeData42
  Scope3 : Scope
      settings: SaveName=ScopeData45
  Subsystem : Subsystem
  To Workspace1 : ToWorkspace  VariableName=CtestB  SampleTime=IMU_DT
  To Workspace2 : ToWorkspace  VariableName=CtestA  SampleTime=IMU_DT
  To Workspace6 : ToWorkspace  VariableName=QAp  SampleTime=IMU_DT
  Trigonometric Function1 : Trigonometry
  Trigonometric Function2 : Trigonometry  Operator=cos
  YAW CMD : Subsystem
  dcm_b_to_track : Outport
  DCM_local_to_track : Outport  Port=2
  yaw : Outport  Port=3
  yawCmd : Outport  Port=4
  wires:
  Constant1/1 -> MATLAB Function/9(C33)
  Constant/1 -> MATLAB Function/3(C13), MATLAB Function/6(C23), MATLAB Function/7(C31), MATLAB Function/8(C32)
  Trigonometric Function2/1 -> MATLAB Function/5(C22), MATLAB Function/1(C11)
  Trigonometric Function1/1 -> Gain1/1, Gain/1
  Gain/1 -> MATLAB Function/4(C21)
  Product/1 -> To Workspace2/1, dcm_b_to_track/1, Scope2/1
  Subsystem/2(dcm_c2b) -> Permute Dimensions/1, Scope3/1
  Subsystem/1(angles) -> Demux1/1
  MATLAB Function/1(R) -> To Workspace1/1, Product/1, DCM_local_to_track/1, Scope1/1
  Gain1/1 -> MATLAB Function/2(C12)
  Permute Dimensions/1 -> Product/2
  Q/1 -> To Workspace6/1, LPF/1(quat)
  LPF/1(qout) -> Subsystem/1(quat)
  V/1 -> YAW CMD/1(v)
  Gain2/1 -> yawCmd/1
  Demux1/3 -> yaw/1
  YAW CMD/1(yawcmd) -> Gain2/1, Trigonometric Function1/1, Trigonometric Function2/1

== system drone/Flight Hardware/control/Autopilot/Command Frame Translation ==
  A_cmd : Inport
  A_meas : Inport  Port=2
  Dcm_b_to_track : Inport  Port=3
  Dcm_local_to_track : Inport  Port=4
  Demux : Demux  Outputs=3
  Demux1 : Demux  Outputs=3
  Product : Product  Multiplication=Matrix(*)
  Product1 : Product  Multiplication=Matrix(*)
  Scope{1..6} (6 alike) : Scope
      Scope1 settings: TimeRange=50  YMin=0  YMax=35  SaveName=ScopeData30
      Scope2 settings: TimeRange=50  YMin=0  YMax=35  SaveName=ScopeData34
      Scope3 settings: TimeRange=20  YMin=0  YMax=10  SaveName=ScopeData24
      Scope4 settings: TimeRange=50  YMin=0  YMax=35  SaveName=ScopeData78
      Scope5 settings: TimeRange=50  YMin=0  YMax=35  SaveName=ScopeData79
      Scope6 settings: TimeRange=20  YMin=0  YMax=10  SaveName=ScopeData85
  To Workspace2 : ToWorkspace  VariableName=AccelAp  SampleTime=IMU_DT
  Ac_in : Outport
  Am_in : Outport  Port=2
  Ac_x : Outport  Port=3
  Am_x : Outport  Port=4
  wires:
  Demux/1 -> Scope6/1, Ac_in/1
  Demux1/1 -> Scope5/1, Am_in/1
  Demux/2 -> Ac_x/1
  Demux1/2 -> Scope4/1, Am_x/1
  A_cmd/1 -> Product/2
  Dcm_local_to_track/1 -> Product/1
  Product/1 -> Scope3/1, Demux/1
  Dcm_b_to_track/1 -> Product1/1
  A_meas/1 -> To Workspace2/1, Scope1/1, Product1/2
  Product1/1 -> Demux1/1

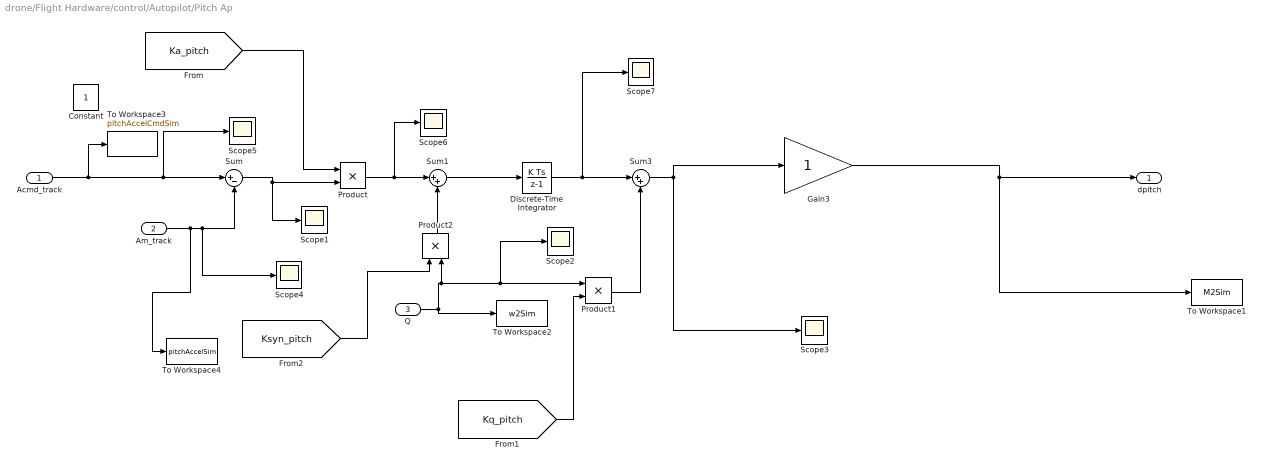
== system drone/Flight Hardware/control/Autopilot/Pitch Ap ==
  Acmd_track : Inport
  Am_track : Inport  Port=2
  Q : Inport  Port=3
  Constant : Constant
  Discrete-Time Integrator : DiscreteIntegrator  InitialConditionSetting=State (most efficient)  SampleTime=-1
  Gain3 : Gain
  Product : Product
  Product1 : Product
  Product2 : Product
  Scope{1..7} (7 alike) : Scope
      Scope1 settings: TimeRange=80  YMin=-0.015  YMax=0.01  SaveName=ScopeData15
      Scope2 settings: TimeRange=80  YMin=0  YMax=0.05  SaveName=ScopeData48
      Scope3 settings: TimeRange=50  YMin=-0.13  YMax=0.02  SaveName=ScopeData12
      Scope4 settings: TimeRange=20  YMin=-40  YMax=40  SaveName=ScopeData25
      Scope5 settings: TimeRange=80  YMin=-70000  YMax=0  SaveName=ScopeData64
      Scope6 settings: TimeRange=50  YMin=-0.25  YMax=3.75  SaveName=ScopeData69
      Scope7 settings: TimeRange=50  YMin=-2.25  YMax=1.5  SaveName=ScopeData70
  Sum : Sum  Inputs=|+-
  Sum1 : Sum  Inputs=|++
  Sum3 : Sum  Inputs=|++
  To Workspace1 : ToWorkspace  VariableName=M2Sim  SampleTime=-1
  To Workspace2 : ToWorkspace  VariableName=w2Sim  SampleTime=-1
  To Workspace3 : ToWorkspace  VariableName=pitchAccelCmdSim  SampleTime=-1
  To Workspace4 : ToWorkspace  VariableName=pitchAccelSim  SampleTime=-1
  dpitch : Outport
  wires:
  Am_track/1 -> To Workspace4/1, Sum/2, Scope4/1
  Product2/1 -> Sum1/2
  Sum1/1 -> Discrete-Time Integrator/1
  Product/1 -> Scope6/1, Sum1/1
  Discrete-Time Integrator/1 -> Scope7/1, Sum3/1
  Product1/1 -> Sum3/2
  Sum3/1 -> Gain3/1, Scope3/1
  Gain3/1 -> To Workspace1/1, dpitch/1
  [Ka_pitch] -> Product/1
  [Kq_pitch] -> Product1/2
  Q/1 -> Product2/2, Scope2/1, Product1/1, To Workspace2/1
  [Ksyn_pitch] -> Product2/1
  Acmd_track/1 -> To Workspace3/1, Sum/1, Scope5/1
  Sum/1 -> Product/2, Scope1/1
